simulink model "Hyped_sm"  (R2019a)
settings: Solver=FixedStepDiscrete  StartTime=0.0  StopTime=10.0  FixedStep=1  RelTol=1e-3
settings Model: Creator=s1449365  LastModifiedBy=s1449365
settings DataIOCC: SaveOutput=off  SignalLogging=off  DSMLogging=off  SaveTime=off  ReturnWorkspaceOutputs=off

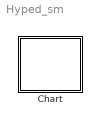
== system Hyped_sm ==
  Chart : Stateflow chart  BlockKeywords=__PRM__SERIALIZED__DATA__:Stateflow Chart,Stateflow Diagram  TreatAsAtomicUnit=on

== stateflow chart Hyped_sm/Chart ==
  state EmergencyBraking
  state FailureStopped
  state Finished
  state Idle
  state Calibrating
  state Ready
  state Accelerating
  state Exiting
  state NominalBraking
  state RunComplete
  FailureStopped -> Idle : [checkReset() == true]
  EmergencyBraking -> FailureStopped : [checkVelocityZeroReached() == true]
  Idle -> EmergencyBraking [order 1] : [checkTelemetryCriticalFailure() == true]
  NominalBraking -> EmergencyBraking [order 1] : [CheckCriticalFailure() == true]
  Accelerating -> EmergencyBraking [order 1] : [CheckCriticalFailure() == true]
  RunComplete -> FailureStopped [order 1] : [CheckCriticalFailure() == true]
  Exiting -> FailureStopped [order 1] : [CheckCriticalFailure() == true]
  Calibrating -> EmergencyBraking [order 1] : [CheckCriticalFailure() == true]
  Ready -> EmergencyBraking [order 1] : [CheckCriticalFailure() == true]
  (default) -> Idle
  Exiting -> Finished [order 2] : [checkFinish() == true]
  Finished -> Idle : [checkReset() == true]
  Accelerating -> NominalBraking [order 2] : [checkTimer() == true]
  RunComplete -> Exiting [order 2] : [checkOnExit() == true]
  Idle -> Calibrating [order 2] : [CheckInitialised() == true]
  Calibrating -> Ready [order 2] : [checkSystemsChecked() == true]
  Ready -> Accelerating [order 2] : [checkOnStart() == true]
  Accelerating -> NominalBraking [order 3] : [checkMaxDIstanceReached() == true]
  NominalBraking -> RunComplete [order 2] : [checkVelocityZeroReached() == true]
